simulink model "model"  (R2013a)
settings: Solver=ode45  StartTime=0.0  StopTime=10.0  MaxStep=0.01  RelTol=1e-3
values from neighbouring files (symbols this model uses):
  d = 0    [calkujacy.m]
  k = 3    [calkujacy.m]    (also in lab3.m = 1)
  T = 2    [calkujacy.m]    (also in lab3.m)
settings Model: Creator=Dawid Perdek  LastModifiedBy=Dawid Perdek

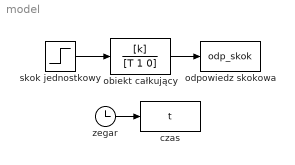
== system model ==
  czas : ToWorkspace  VariableName=t  SampleTime=-1
  obiekt całkujący : TransferFcn  Numerator=[k]  Denominator=[T 1 0]
  odpowiedz skokowa : ToWorkspace  VariableName=odp_skok  SampleTime=-1
  skok jednostkowy : Step  Time=d  SampleTime=0
  zegar : Clock
  wires:
  zegar/1 -> czas/1
  skok jednostkowy/1 -> obiekt całkujący/1
  obiekt całkujący/1 -> odpowiedz skokowa/1
